simulink model "step1"  (R2018b)
settings: Solver=VariableStepAuto  StartTime=0.0  StopTime=1  RelTol=1e-3
libraries: simulink_extras x1
settings Model: Creator=ali  LastModifiedBy=Ali

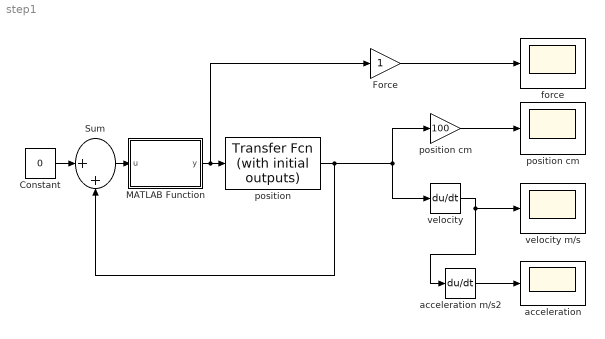
== system step1 ==
  Constant : Constant  Value=0
  Force : Gain
  MATLAB Function : MATLAB Function  TreatAsAtomicUnit=on
  Sum : Sum  Inputs=|++
  "acceleration " : Scope
  acceleration m/s2 : Derivative
  "force " : Scope
  position : simulink_extras/Additional Linear/Transfer Fcn (with initial outputs)  N=[1]  D=[1 10 100]  Y0=0  U0=0.4
  position cm : Gain  Gain=100
  "position cm " : Scope
  velocity : Derivative
  "velocity m/s " : Scope
  wires:
  MATLAB Function/1(y) -> Force/1, position/1
  position/1 -> velocity/1, position cm/1, Sum/2
  velocity/1 -> acceleration m/s2/1, "velocity m/s "/1
  acceleration m/s2/1 -> "acceleration "/1
  position cm/1 -> "position cm "/1
  Constant/1 -> Sum/1
  Sum/1 -> MATLAB Function/1(u)
  Force/1 -> "force "/1

== matlab function step1/MATLAB Function ==
  data: u input; y output
function y = fcn(u)
if u>=0
    y=-1;
else
    y=1;
end
